simulink model "week3_vendingMachine"  (R2020b)
settings: Solver=VariableStepAuto  StartTime=0.0  StopTime=200  RelTol=1e-3
settings Model: Creator=hp  LastModifiedBy=hp

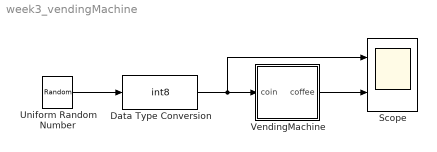
== system week3_vendingMachine ==
  Data Type Conversion : DataTypeConversion  OutDataTypeStr=int8  RndMeth=Nearest  SaturateOnIntegerOverflow=on
  Scope : Scope  NumInputPorts=2
  Uniform Random Number : UniformRandomNumber  Minimum=0  Maximum=2  Seed=337  SampleTime=10
  VendingMachine : Stateflow chart  TreatAsAtomicUnit=on
  wires:
  Data Type Conversion/1 -> VendingMachine/1(coin), Scope/1
  Uniform Random Number/1 -> Data Type Conversion/1
  VendingMachine/1(coffee) -> Scope/2

== stateflow chart week3_vendingMachine/VendingMachine ==
  settings: stateMachineType=MEALY_MACHINE  initializeOutput=1
  state state1
  state state2l
  state state3
  (default) -> state1
  state1 -> state2l [order 1] : [coin==1]{coffee=0}
  state2l -> state1 [order 2] : [coin==2]{coffee=1}
  state3 -> state1 [order 1] : [coin==1]{coffee=1}
  state1 -> state3 [order 2] : [coin==2]{coffee=0}
  state2l -> state3 [order 1] : [coin==1]{coffee=0}
  state3 -> state2l [order 2] : [coin==2]{coffee=1}
  data: coin input int8; coffee output double
